simulink model "PMT_AI_Env_Version0_MatlabRL"  (R2025a)
settings: Solver=ode4  StartTime=0.0  StopTime=10.0  FixedStep=0.001  RelTol=1e-3
libraries: slpidlib x1, rllib x1
settings Model: Creator=30623  LastModifiedBy=30623

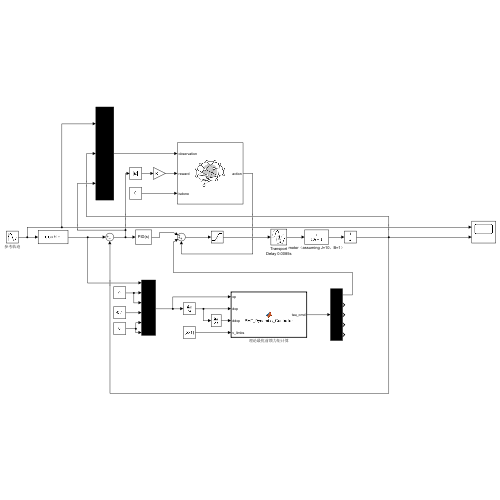
[thumbnail: Simulink's stored preview of the top-level diagram]
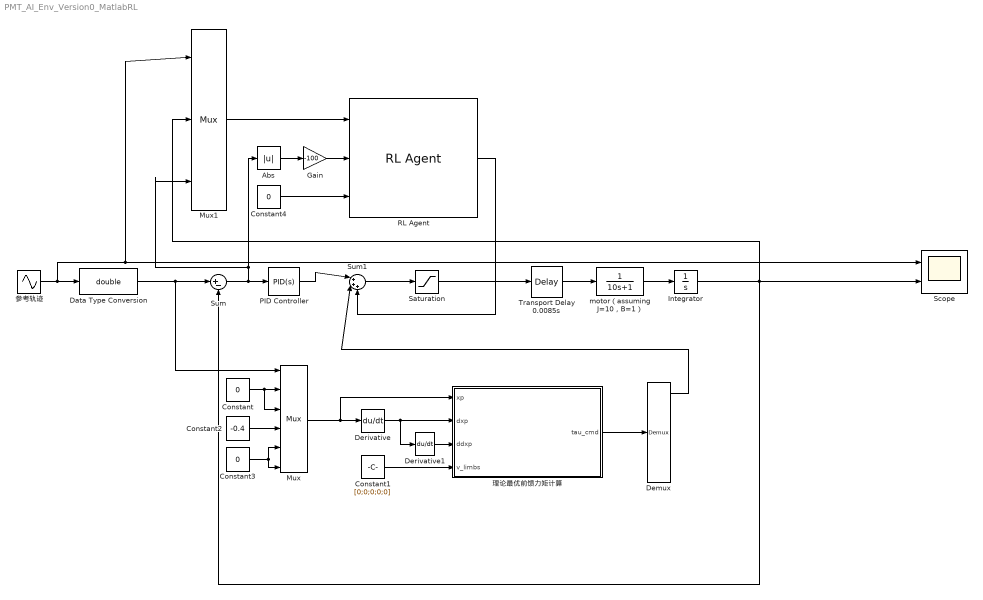
== system PMT_AI_Env_Version0_MatlabRL ==
  Abs : Abs  SaturateOnIntegerOverflow=off
  Constant : Constant  Value=0
  Constant1 : Constant  Value=[0;0;0;0;0]
  Constant2 : Constant  Value=-0.4
  Constant3 : Constant  Value=0
  Constant4 : Constant  Value=0
  Data Type Conversion : DataTypeConversion  OutDataTypeStr=double  SaturateOnIntegerOverflow=off  RndMeth=Floor
  Demux : Demux  Outputs=5
  Derivative : Derivative
  Derivative1 : Derivative
  Gain : Gain  Gain=-100
  Integrator : Integrator
  Mux : Mux  Inputs=6
  Mux1 : Mux  Inputs=3
  PID Controller : slpidlib/PID Controller  Controller=PID  Form=Parallel  TimeDomain=Continuous-time  UseExternalTs=off  SampleTime=-1  IntegratorMethod=Forward Euler  FilterMethod=Forward Euler  ControllerParametersSource=internal  P=1  I=1  UseKiTs=off  D=0  UseExternalDerivativeSource=off  N=100  UseFilter=on  TunerSelectOption=Transfer Function Based (PID Tuner App)  InitialConditionSource=internal  InitialConditionForIntegrator=0  InitialConditionForFilter=0  DifferentiatorICPrevScaledInput=0  ExternalReset=none  TrackingMode=off  Kt=1  LimitOutput=off  SatLimitsSource=internal  UpperSaturationLimit=inf  LowerSaturationLimit=-inf  LinearizeAsGain=on  AntiWindupMode=none  Kb=1  LimitIntegrator=off  UpperIntegratorSaturationLimit=inf  LowerIntegratorSaturationLimit=-inf  POutMin=[]  POutMax=[]  IOutMin=[]  IOutMax=[]  DOutMin=[]  DOutMax=[]  NOutMin=[]  NOutMax=[]  SumOutMin=[]  SumOutMax=[]  SaturationOutMin=[]  SaturationOutMax=[]  PParamMin=[]  PParamMax=[]  IParamMin=[]  IParamMax=[]  DParamMin=[]  DParamMax=[]  NParamMin=[]  NParamMax=[]  KbParamMin=[]  KbParamMax=[]  KtParamMin=[]  KtParamMax=[]  KbOutMin=[]  KbOutMax=[]  KtOutMin=[]  KtOutMax=[]  IntegratorOutMin=[]  IntegratorOutMax=[]  FilterOutMin=[]  FilterOutMax=[]  SumI1OutMin=[]  SumI1OutMax=[]  SumI2OutMin=[]  SumI2OutMax=[]  SumI3OutMin=[]  SumI3OutMax=[]  SumI4OutMin=[]  SumI4OutMax=[]  SumDOutMin=[]  SumDOutMax=[]  DifferentiatorOutMin=[]  DifferentiatorOutMax=[]  FilterDiffOutCoefMin=[]  FilterDiffOutCoefMax=[]  ReciprocalOutMin=[]  ReciprocalOutMax=[]  SumDenOutMin=[]  SumDenOutMax=[]  SumNumOutMin=[]  SumNumOutMax=[]  DivideOutMin=[]  DivideOutMax=[]  UdiffTsProdOutMin=[]  UdiffTsProdOutMax=[]  NTsProdOutMin=[]  NTsProdOutMax=[]  UintegralTsProdOutMin=[]  UintegralTsProdOutMax=[]  UngainTsProdOutMin=[]  UngainTsProdOutMax=[]  ClampingZeroOutDataTypeStr=Inherit: Inherit via back propagation  ClampingZeroOutMin=[]  ClampingZeroOutMax=[]  FilterDenConstantOutDataTypeStr=Inherit: Inherit via back propagation  FilterDenConstantOutMin=[]  FilterDenConstantOutMax=[]  PCopyOutDataTypeStr=Inherit: Inherit via back propagation  PCopyOutMin=[]  PCopyOutMax=[]  NCopyOutDataTypeStr=Inherit: Inherit via back propagation  NCopyOutMin=[]  NCopyOutMax=[]  IntegratorContinuousStateAttributes=''  IntegratorStateMustResolveToSignalObject=off  IntegratorRTWStateStorageClass=Auto  FilterContinuousStateAttributes=''  FilterStateMustResolveToSignalObject=off  FilterRTWStateStorageClass=Auto  ParallelPVariant=InternalParameters  IdealPVariant=Disabled  IVariant=InternalParameters  DVariant=InternalParameters  IntegratorVariant=Continuous  SatVariant=Disabled  AWVariant=Passthrough  PCopyVariant=Disabled  TRVariant=Disabled  FdbkBlocksVariant=Forward  IdealPFdbkVariant=Disabled  SatFdbkVariant=Disabled  DerivativeFilterVariant=ContFilter  NVariant=InternalParameters  NCopyVariant=Disabled  FilterICVariant=InternalICsFilter  IntegratorICVariant=InternalICs  ExternalResetVariant=Disabled  TRSumVariant=Passthrough  SumFdbkVariant=Disabled  SumVariant=Sum_PID  TsampFilterVariant=InternalTs  TsampNgainVariant=Passthrough  TsampIntegralVariant=Disabled_SignalSpec  ExternalSaturationOutDataTypeStr=Inherit: Same as second input  DerivativeSourceVariant=ErrorSignal  PreIntVariant=InternalPreInt
  RL Agent : rllib/RL Agent  Agent=agentObj  ExternalActionAsInput=off  ProvideLastAction=off  ProvideCumRwd=off  TreatAsDirectFeedthrough=on  UseStrictObservationDataTypes=off
  Saturation : Saturate  UpperLimit=500  LowerLimit=-500
  Scope : Scope  NumInputPorts=2
      settings: ActiveDisplayYMinimum=-1409.4591866243368  ActiveDisplayYMaximum=2153.1031709558697
  Sum : Sum  Inputs=|+-
  Sum1 : Sum  Inputs=|+++
  Transport Delay 0.0085s : TransportDelay  DelayTime=0.00875
  motor（assuming J=10，B=1） : TransferFcn  Denominator=[10 1]
  参考轨迹 : Sin  Amplitude=0.05  Frequency=2  SampleTime=0
  理论最优前馈力矩计算 : MATLAB Function  TreatAsAtomicUnit=on
  wires:
  Transport Delay 0.0085s/1 -> motor（assuming J=10，B=1）/1
  Data Type Conversion/1 -> Mux/1, Sum/1
  Sum/1 -> Abs/1, Mux1/3, PID Controller/1
  motor（assuming J=10，B=1）/1 -> Integrator/1
  Integrator/1 -> Mux1/2, Sum/2, Scope/2
  PID Controller/1 -> Sum1/1
  Constant/1 -> Mux/3, Mux/2
  Mux/1 -> 理论最优前馈力矩计算/1(xp), Derivative/1
  Derivative/1 -> Derivative1/1, 理论最优前馈力矩计算/2(dxp)
  Derivative1/1 -> 理论最优前馈力矩计算/3(ddxp)
  Constant1/1 -> 理论最优前馈力矩计算/4(v_limbs)
  理论最优前馈力矩计算/1(tau_cmd) -> Demux/1
  Demux/1 -> Sum1/2
  参考轨迹/1 -> Mux1/1, Scope/1, Data Type Conversion/1
  Constant2/1 -> Mux/4
  Constant3/1 -> Mux/6, Mux/5
  Sum1/1 -> Saturation/1
  Saturation/1 -> Transport Delay 0.0085s/1
  RL Agent/1 -> Sum1/3
  Mux1/1 -> RL Agent/1
  Abs/1 -> Gain/1
  Gain/1 -> RL Agent/2
  Constant4/1 -> RL Agent/3

== matlab function PMT_AI_Env_Version0_MatlabRL/理论最优前馈力矩计算 ==
  data: xp input; tau_cmd output; dxp input; ddxp input; v_limbs input
%理论最优前馈力矩计算
function tau_cmd = PMT_Dynamics_Controller(xp, dxp, ddxp, v_limbs)
    % 输入: 
    % xp: [x, y, z, phi, theta]' 动平台位姿 (T&T angles)
    % dxp: [v_x, v_y, v_z, w_x, w_y, w_z]' 动平台速度 
    % ddxp: [a_x, a_y, a_z, dw_x, dw_y, dw_z]' 动平台加速度 
    % v_limbs: [v1, v2, v3, v4, v5]' 五个驱动支链的实际线速度 (用于计算摩擦力) 
    % 输出:
    % tau_cmd: [tau1, tau2, tau3, tau4, tau5]' 五个伺服电机的目标前馈力矩
    % 定义反对称矩阵算子 S(v)，用于计算叉乘 
    S = @(v) [0, -v(3), v(2); v(3), 0, -v(1); -v(2), v(1), 0];
    
    %% 1. 物理与几何参数化
    % 动平台真实辨识惯性参数 (摘自解老师论文 Table 2) 
    m_p = 45.32; 
    mp_es = 8.384; 
    I_xx = 6.24e-4; I_yy = 6.24e-4; I_zz = 1.03e-4;
    I_p_matrix = diag([I_xx, I_yy, I_zz]); % 忽略极小的耦合项 
    g_vec = [0; 0; -9.81]; 
    
    % 驱动支链真实辨识摩擦力参数 (摘自论文 Table 1: [Tc, Ts, vs, Bv]) 
    Fric_Params = [
        186.21, 291.52, -1.87, 3.027; % Limb 1
        244.34, 372.97,  1.26, 3.766; % Limb 2
        187.89, 273.38,  1.35, 3.006; % Limb 3
        226.99, 314.07,  1.30, 3.489; % Limb 4
        224.82, 312.41,  2.69, 2.696  % Limb 5
    ];
    
    % 虚拟几何参数 (因原论文未公开，用于 DRL 环境预研构建)
    R_b = 0.5; % 基座分布半径 0.5m
    b = [
        0,  R_b*cos(pi/4), R_b*cos(3*pi/4), R_b*cos(5*pi/4), R_b*cos(7*pi/4);
        0,  R_b*sin(pi/4), R_b*sin(3*pi/4), R_b*sin(5*pi/4), R_b*sin(7*pi/4);
        0,  0,             0,               0,               0
    ];
    
    R_p = 0.15; % 动平台铰链分布半径 0.15m
    H_tool = -0.1; % 刀尖到平台铰链面的 Z 向距离
    p_local = [
        0,       R_p*cos(pi/4), R_p*cos(3*pi/4), R_p*cos(5*pi/4), R_p*cos(7*pi/4);
        0,       R_p*sin(pi/4), R_p*sin(3*pi/4), R_p*sin(5*pi/4), R_p*sin(7*pi/4);
        H_tool,  H_tool,        H_tool,          H_tool,          H_tool
    ];
    
    %% 2. 运动学正解与雅可比矩阵构建 
    % (1) 计算旋转矩阵 R (基于 T&T angles, Eq. A-1) 
    phi = xp(4); theta = xp(5);
    p_vec = [cos(phi)*sin(theta); sin(phi)*sin(theta); cos(theta)];
    
    % 依据原论文的投影法生成正交旋转矩阵 R 
    O_B1 = b(:,1); 
    n_vec = cross(O_B1, p_vec); 
    if norm(n_vec) < 1e-6
        n_vec = [1;0;0]; % 奇异保护
    else
        n_vec = n_vec / norm(n_vec);
    end
    o_vec = cross(p_vec, n_vec);
    R = [n_vec, o_vec, p_vec];
    
    % (2) 运动传递雅可比 J_t (5x6 矩阵) 
    J_t = zeros(5, 6); 
    l_unit_all = zeros(3, 5); % 保存单位方向向量备用
    L_all = zeros(1, 5);      % 保存支链长度备用
    p_global_all = zeros(3, 5); % 保存全局坐标备用
    for i = 1:5
        p_i_global = R * p_local(:, i); % Eq. A-2 
        p_global_all(:, i) = p_i_global;
        
        l_vec = (xp(1:3) + p_i_global) - b(:, i); % Eq. A-3 
        L_i = norm(l_vec);
        L_all(i) = L_i;
        l_unit = l_vec / L_i; % Eq. A-3 
        l_unit_all(:, i) = l_unit;
        
        J_t(i, :) = [l_unit', (cross(p_i_global, l_unit))']; % 组装 J_t 
    end
    
    % (3) 约束雅可比 J_c (1x6 矩阵，第一条 SPR 支链提供的一维约束) 
    J_c = [n_vec', (L_all(1) * cross(n_vec, l_unit_all(:,1)) + cross(p_global_all(:,1), n_vec))'];
    % 组装完整满秩雅可比矩阵 J_a (6x6 矩阵) 
    J_a = [J_t; J_c]; 
    
    %% 3. 动力学受力分析 (附录 A.2 解老师用到了虚功原理) 
    % (1) 动平台惯性力和重力 F_p (Eq. A-12) 
    w_p = dxp(4:6);   % 角速度
    dw_p = ddxp(4:6); % 角加速度
    a_c = ddxp(1:3);  % 线加速度
    
    F_p_trans = m_p * g_vec - m_p * a_c; 
    F_p_rot = -I_p_matrix * dw_p - cross(w_p, I_p_matrix * w_p);
    F_p = [F_p_trans; F_p_rot]; % 6x1 向量
    
    % (2) 支链惯性力简化 (为提高仿真速度，此处将支链质量等效附加到平台上)
    F_limbs_total = zeros(6, 1); 
    
    %% 4. 虚功反解理论刚体力矩 
    % 求解: J_a' * [tau_ideal; F_constraint] = - F_p 
   Tau_and_Constraint = pinv(J_a') * (-F_p - F_limbs_total);
    tau_ideal = Tau_and_Constraint(1:5); % 提取前5个主动电机的理论力矩
    
    %% 5. Stribeck 非线性摩擦力补偿 (Eq. 4) 
    f_friction = zeros(5, 1);
    for i = 1:5
        v = v_limbs(i);
        Tc = Fric_Params(i, 1);
        Ts = Fric_Params(i, 2);
        vs = Fric_Params(i, 3);
        Bv = Fric_Params(i, 4);
       
        f_friction(i) = (Tc + (Ts - Tc) * exp(-(v/vs)^2)) * sign(v) + Bv * v; 
    end
    
    %% 6. 输出最终前馈力矩指令 
    tau_cmd = tau_ideal + f_friction;
end
